simulink model "leadcontrolla"  (R2023a)
settings: Solver=ode4  StartTime=0.0  StopTime=Te - Ts + Tt  FixedStep=0.002  RelTol=1e-3  EnableMultiTasking=on
PostLoadFcn:
  | qc_set_target_type(getConfigSet(bdroot, 'QUARC Default Target Configuration'));
values from neighbouring files (symbols this model uses):
  phaseRand = 2*pi*rand(1,N)    [Init.m]    (also in phiOffsetNoDriftData.mat = [0.35156011067 5.13245242595 3.32331786907 4.36273324053 1.3; rootLocusController.mat = [4.29591163885 0.829901686668 4.54101220871 0.693371368168 0)
  wc = 150    [Init.m]    (also in phiOffsetNoDriftData.mat; rootLocusController.mat)
  wf = [1:N]*wr    [Init.m]    (also in phiOffsetNoDriftData.mat = [0.418879020479 0.837758040957 1.25663706144 1.67551608191 2; rootLocusController.mat = [0.418879020479 0.837758040957 1.25663706144 1.67551608191 2)
undefined symbols (not defined in the file or in its folder): HIL
libraries: quarc_library x5, cstblocks x3
settings Model: SimulationMode=external  ExtModeTrigDuration=10000  Creator=MLevis  LastModifiedBy=quarc_user
settings SolverCC: AlgebraicLoopSolver=TrustRegion  PositivePriorityOrder=on  AutoInsertRateTranBlk=on
settings DataIOCC: LimitDataPoints=on  SaveFormat=Array  SignalLoggingSaveFormat=ModelDataLogs  ReturnWorkspaceOutputs=off
settings OptimizationCC: ExpressionDepthLimit=2147483647  InitFltsAndDblsToZero=on
settings DebuggingCC: SaveWithParameterizedLinksMsg=none  UnderspecifiedInitializationDetection=Classic  MergeDetectMultiDrivingBlocksExec=none  SolverPrmCheckMsg=warning  MultiTaskDSMMsg=warning  MultiTaskCondExecSysMsg=none  FcnCallInpInsideContextMsg=warning  UnconnectedInputMsg=warning  UnconnectedOutputMsg=warning  UnconnectedLineMsg=warning  StateNameClashWarn=warning  SFUnexpectedBacktrackingDiag=warning  SFNoUnconditionalDefaultTransitionDiag=warning  SFExecutionAtInitializationDiag=none  ArithmeticOperatorsInVariantConditions=warning
settings ModelReferenceCC: EnableRefExpFcnMdlSchedulingChecks=on  PropagateSignalLabelsOutOfModel=off
settings SFSimCC: SimUseLocalCustomCode=off  CustomCodeUndefinedFunction=UseInterfaceOnly
settings RTWCC: Description=QUARC Win64 Target Using Toolchain  SystemTargetFile=quarc_win64.tlc  TemplateMakefile=quarc_default_tmf  RTWUseLocalCustomCode=off  Toolchain=QUARC win64 | nmake (64-bit Windows)  BuildConfiguration=Faster Runs  DLArmComputeVersion=19.05
settings CodeAppCC: StateflowObjectComments=on
settings STFCustomTargetCC: TargetLangStandard=C89/C90 (ANSI)  SystemTargetFile=quarc_win64.tlc
settings GRTTargetCC: TargetLangStandard=C89/C90 (ANSI)  ParMdlRefBuildCompliant=off  CompOptLevelCompliant=off  CombineOutputUpdateFcns=off  MatFileLogging=off  CPPClassGenCompliant=off  GRTInterface=on  ExtMode=on  ExtModeMexFile=quarc_comm
settings ConfigComp: CovMetricSettings=dw  CovSaveCumulativeToWorkspaceVar=on  CovSaveSingleToWorkspaceVar=on  CovExternalEMLEnable=off

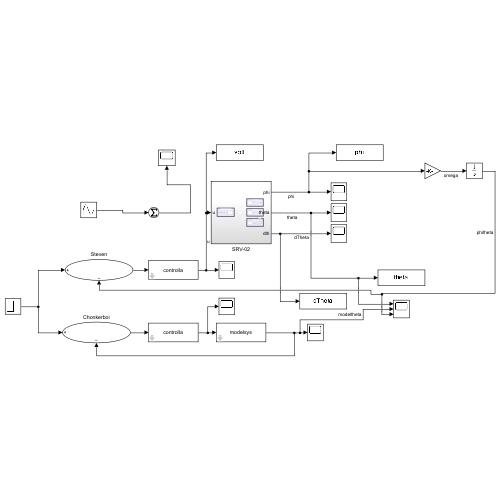
[thumbnail: Simulink's stored preview of the top-level diagram]
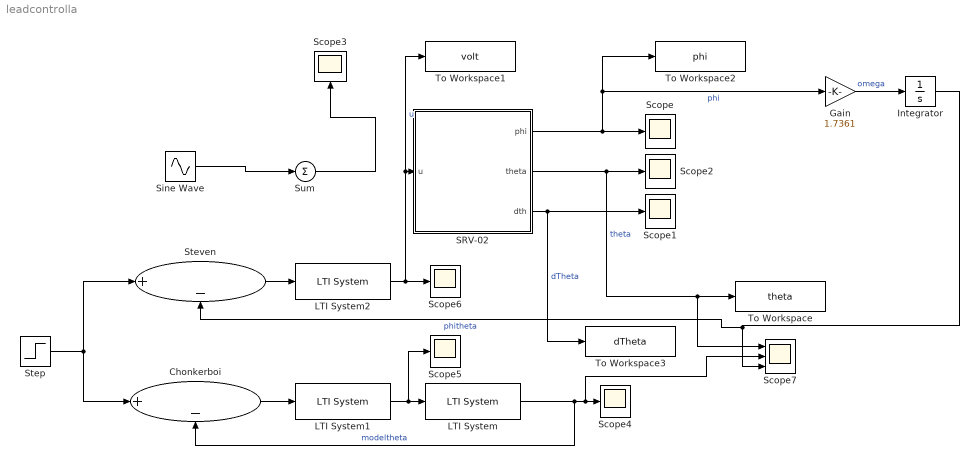
== system leadcontrolla ==
  Chonkerboi : Sum  Inputs=|+-
  Gain : Gain  Gain=1.7361
  Integrator : Integrator
  LTI System : cstblocks/LTI System  sys=modelsys  IC=[]
  LTI System1 : cstblocks/LTI System  sys=controlla  IC=[]
  LTI System2 : cstblocks/LTI System  sys=controlla  IC=[]
  SRV-02 : Subsystem
  Scope{,1..6} (7 alike) : Scope
  Scope7 : Scope  NumInputPorts=3
  Sine Wave : Sin  Amplitude=0.2  Frequency=wf  Phase=phaseRand  SampleTime=0
  Step : Step  SampleTime=0
  Steven : Sum  Inputs=|+-
  Sum : Sum  Inputs=+
  To Workspace : ToWorkspace  VariableName=theta  SampleTime=-1
      settings: MaxDataPoints=Te/Ts
  To Workspace1 : ToWorkspace  VariableName=volt  SampleTime=-1
      settings: MaxDataPoints=Te/Ts
  To Workspace2 : ToWorkspace  VariableName=phi  SampleTime=-1
      settings: MaxDataPoints=Te/Ts
  To Workspace3 : ToWorkspace  VariableName=dTheta  SampleTime=-1
      settings: MaxDataPoints=Te/Ts
  wires:
  SRV-02/1(phi) -> Gain/1, To Workspace2/1, Scope/1  "phi"
  SRV-02/3(dth) -> To Workspace3/1, Scope1/1  "dTheta"
  SRV-02/2(theta) -> Scope7/1, To Workspace/1, Scope2/1  "theta"
  Sine Wave/1 -> Sum/1
  Sum/1 -> Scope3/1
  LTI System1/1 -> Scope5/1, LTI System/1
  LTI System/1 -> Chonkerboi/2, Scope7/2, Scope4/1  "modeltheta"
  Chonkerboi/1 -> LTI System1/1
  Step/1 -> Chonkerboi/1, Steven/1
  Steven/1 -> LTI System2/1
  LTI System2/1 -> To Workspace1/1, SRV-02/1(u), Scope6/1  "u"
  Gain/1 -> Integrator/1  "omega"
  Integrator/1 -> Steven/2, Scope7/3  "phitheta"

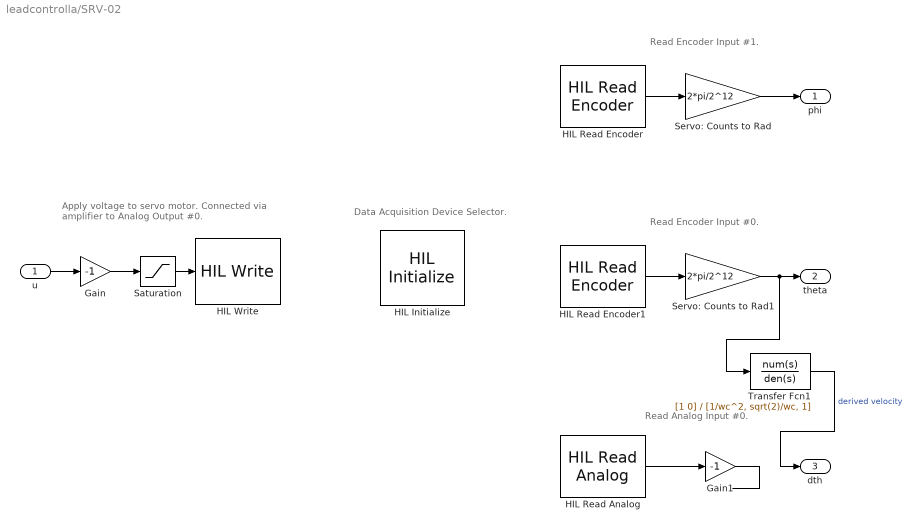
== system leadcontrolla/SRV-02 ==
  note: Apply voltage to servo motor.
      | Connected via amplifier to Analog Output #0.
  note: Read Analog Input #0.
  note: Read Encoder Input #1.
  note: Data Acquisition Device Selector.
  note: Read Encoder Input #0.
  u : Inport
  Gain : Gain  Gain=-1
  Gain1 : Gain  Gain=-1
  HIL Initialize : quarc_library/Data Acquisition/Generic/Configuration/HIL Initialize  object_name=HIL-1  board_type=q2_usb  board_number=0  board_options=d0=digital;d1=digital;led=auto;update_rate=normal;decimation=1  exclusive=off  active=off  hardware_clocks=[0]  clock_modes=[]  initial_clock_frequencies=[]  set_clock_params_at_start=off  set_clock_params_at_switch_in=off  set_clock_frequencies_at_start=off  set_clock_frequencies_at_switch_in=off  analog_input_channels=[0:1]  analog_input_configurations=[]  analog_input_maximums=10  analog_input_minimums=-10  set_analog_input_params_at_start=on  set_analog_input_params_at_switch_in=off  analog_output_channels=[0:1]  analog_output_maximums=10  analog_output_minimums=-10  initial_analog_outputs=[0]  final_analog_outputs=[0]  watchdog_analog_outputs=0  set_analog_output_params_at_start=on  set_analog_output_params_at_switch_in=off  set_analog_outputs_at_start=on  set_analog_outputs_at_switch_in=off  set_analog_outputs_at_terminate=on  set_analog_outputs_at_switch_out=off  set_analog_outputs_on_watchdog=off  digital_input_channels=[]  digital_output_channels=[]  digital_output_configuration=[]  initial_digital_outputs=[1]  final_digital_outputs=[1]  watchdog_digital_outputs=[1]  set_digital_output_params_at_start=off  set_digital_output_params_at_switch_in=off  set_digital_outputs_at_start=on  set_digital_outputs_at_switch_in=off  set_digital_outputs_at_terminate=on  set_digital_outputs_at_switch_out=off  set_digital_outputs_on_watchdog=off  encoder_channels=[0:1]  quadrature=[4]  encoder_filter_frequency=[]  initial_encoder_counts=[0]  set_encoder_params_at_start=on  set_encoder_params_at_switch_in=off  set_encoder_counts_at_start=on  set_encoder_counts_at_switch_in=off  pwm_channels=[]  pwm_modes=[0]  pwm_frequency=1/0.020  pwm_configuration=[]  pwm_alignment=[]  pwm_polarity=[]  pwm_leading_deadband=[]  pwm_trailing_deadband=[]  initial_pwm_outputs=[0]  final_pwm_outputs=[0]  watchdog_pwm_outputs=[0]  set_pwm_params_at_start=on  set_pwm_params_at_switch_in=off  set_pwm_outputs_at_start=on  set_pwm_outputs_at_switch_in=off  set_pwm_outputs_at_terminate=on  set_pwm_outputs_at_switch_out=off  set_pwm_outputs_on_watchdog=off  other_output_channels=[]  initial_other_outputs=[]  final_other_outputs=[]  watchdog_other_outputs=[]  set_other_outputs_at_start=off  set_other_outputs_at_switch_in=off  set_other_outputs_at_terminate=off  set_other_outputs_at_switch_out=off  set_other_outputs_on_watchdog=off
  HIL Read Analog : quarc_library/Data Acquisition/Generic/Immediate I//O/HIL Read Analog  object_name=HIL-1  channels=[0]  sample_time=qc_get_step_size  active=on  vector_output=off
  HIL Read Encoder : quarc_library/Data Acquisition/Generic/Immediate I//O/HIL Read Encoder  object_name=HIL-1  channels=1  sample_time=qc_get_step_size  active=on  vector_output=off  data_type_mode=Inherit via back propagation  data_type=double
  HIL Read Encoder1 : quarc_library/Data Acquisition/Generic/Immediate I//O/HIL Read Encoder  object_name=HIL-1  channels=0  sample_time=qc_get_step_size  active=on  vector_output=off  data_type_mode=Inherit via back propagation  data_type=double
  HIL Write : quarc_library/Data Acquisition/Generic/Immediate I//O/HIL Write  Tag=unassigned  object_name=HIL-1  analog_channels=0  pwm_channels=[]  digital_channels=[]  other_channels=[]  sample_time=-1  active=off  vector_input=off
  Saturation : Saturate  UpperLimit=10  LowerLimit=-10
  Servo: Counts to Rad : Gain  Gain=2*pi/2^12
  Servo: Counts to Rad1 : Gain  Gain=2*pi/2^12
  Transfer Fcn1 : TransferFcn  Numerator=[1 0]  Denominator=[1/wc^2, sqrt(2)/wc, 1]  ParameterTunability=Unconstrained
  phi : Outport
  theta : Outport  Port=2
  dth : Outport  Port=3
  wires:
  HIL Read Encoder/1 -> Servo: Counts to Rad/1
  HIL Read Analog/1 -> Gain1/1
  Servo: Counts to Rad/1 -> phi/1
  u/1 -> Gain/1
  Saturation/1 -> HIL Write/1
  Gain/1 -> Saturation/1
  Gain1/1 -> ?
  Servo: Counts to Rad1/1 -> Transfer Fcn1/1, theta/1
  HIL Read Encoder1/1 -> Servo: Counts to Rad1/1
  Transfer Fcn1/1 -> dth/1  "derived velocity"
